simulink model "regulator_discret"  (R2019b)
settings: Solver=VariableStepAuto  StartTime=0.0  StopTime=500  RelTol=1e-3
libraries: cstblocks x1
settings Model: Creator=ialex  LastModifiedBy=ialex

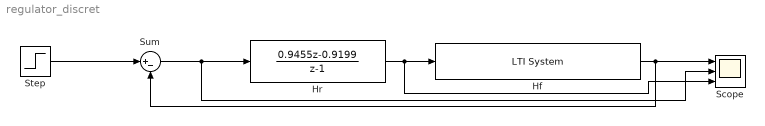
== system regulator_discret ==
  Hf : cstblocks/LTI System  sys=tf(0.5273,[53.3333 1],'ioDelay',12)  IC=[]
  Hr : DiscreteTransferFcn  Numerator=[0.9455 -0.9199]  Denominator=[1 -1]  SampleTime=1
  Scope : Scope  NumInputPorts=3
  Step : Step  Time=0  SampleTime=0
  Sum : Sum  Inputs=|+-
  wires:
  Sum/1 -> Scope/2, Hr/1
  Step/1 -> Sum/1
  Hf/1 -> Sum/2, Scope/1
  Hr/1 -> Scope/3, Hf/1
